simulink model "chap02_75"  (R2013b)
settings: Solver=ode4  StartTime=0.0  StopTime=10.0  FixedStep=0.01  RelTol=1e-3
settings Model: Creator=Administrator  LastModifiedBy=sunzx.fnst
settings DebuggingCC: AlgebraicLoopMsg=error

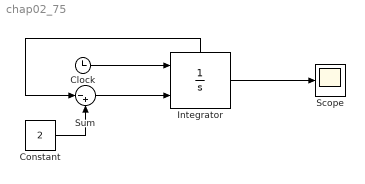
== system chap02_75 ==
  Clock : Clock
  Constant : Constant  Value=2
  Integrator : Integrator  ExternalReset=falling  ShowStatePort=on
  Scope : Scope
  Sum : Sum  Inputs=|-+
  wires:
  Clock/1 -> Integrator/1
  Constant/1 -> Sum/2
  Sum/1 -> Integrator/2
  Integrator/1 -> Scope/1
  Integrator/State -> Sum/1
